simulink model "sampleModel291"  (R2021b)
settings: Solver=VariableStepAuto  StartTime=0.0  StopTime=10.0  RelTol=1e-3
undefined symbols (not defined in the file or in its folder): DiscIntNeverNeededParam
libraries: simulink x16, slpidlib x3
settings Model: Creator=user  LastModifiedBy=user

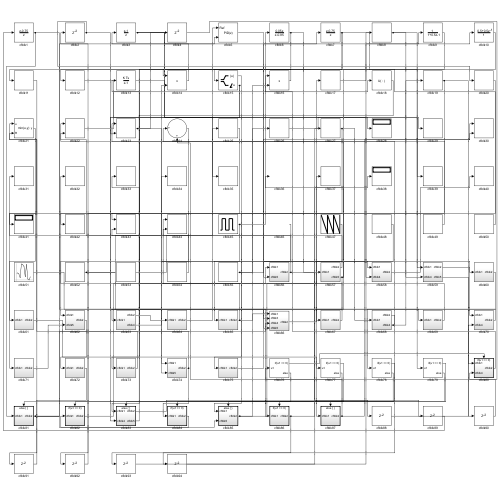
[thumbnail: Simulink's stored preview of the top-level diagram]
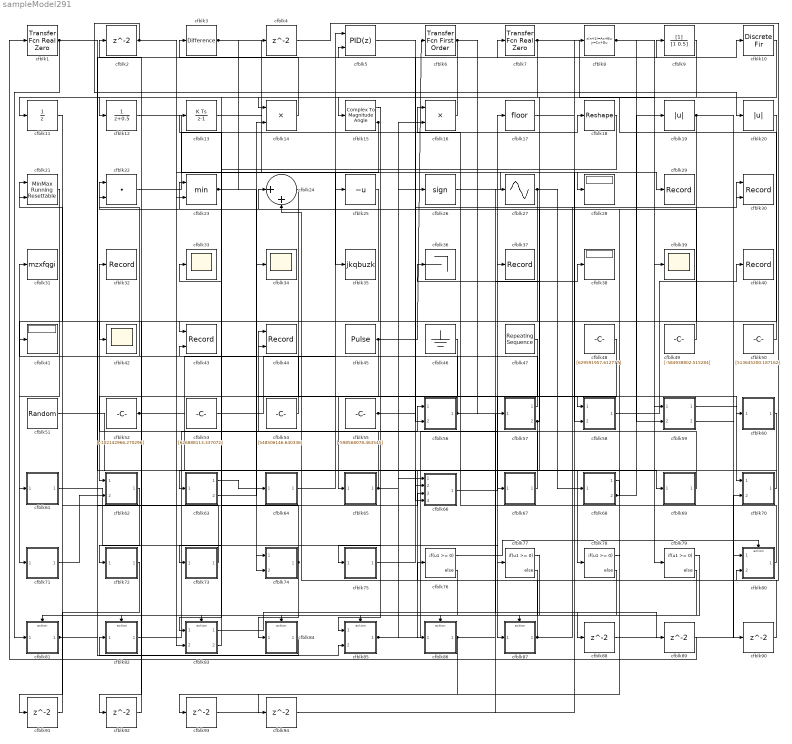
== system sampleModel291 ==
  cfblk1 : simulink/Discrete/Transfer Fcn Real Zero  ZeroZ=0.75  ICPrevInput=0.0  DoSatur=off
      settings: SourceProductBaseCode=SL
  cfblk10 : DiscreteFir  SampleTime=1
  cfblk11 : UnitDelay  HasFrameUpgradeWarning=on
  cfblk12 : DiscreteTransferFcn  SampleTime=1
  cfblk13 : DiscreteIntegrator  ICPrevOutput=DiscIntNeverNeededParam  ICPrevScaledInput=DiscIntNeverNeededParam
  cfblk14 : Product  Inputs=**
  cfblk15 : ComplexToMagnitudeAngle
  cfblk16 : Product
  cfblk17 : Rounding
  cfblk18 : Reshape
  cfblk19 : Abs
  cfblk{2,4,88..94} (9 alike) : Delay  SampleTime=1
  cfblk20 : Abs
  cfblk21 : simulink/Math Operations/MinMax Running Resettable  Function=min  vinit=0.0
  cfblk22 : DotProduct  InputSameDT=on  OutDataTypeStr=Inherit: Inherit via internal rule
  cfblk23 : MinMax  Inputs=2
  cfblk24 : Sum  Inputs=|++
  cfblk25 : UnaryMinus
  cfblk26 : Signum
  cfblk27 : Sin  TimeSource=Use external signal  SampleTime=0
  cfblk28 : Display
  cfblk29 : Record  FileSettingsInternal="{\"entries\":[{\"content\":{\"excelSettings\":{\"content\":{},\"type\":\"Streamout.ExcelSettings\"}},\"type\":\"Streamout.FileSettingStorage\",\"uuid\":\"2b0b6815-d365-4954-8dd6-cb2e8cf74314\"}],\"packageUris\":[\"http://schema.mathworks.com/mf0/streamout_blocks/R2020a\"],\"version\":\"1.0\"}"  SignalsInternal="{\"entries\":[{\"content\":{\"signals\":[{\"content\":{\"blockPath\":[\"sampleModel291/cfblk29\"],\"channel\":[],\"dimensions\":[1],\"domain\":\"sampleModel291/cfblk29\",\"lineColor\":\"#edb120\",\"plots\":[1],\"port\":1,\"sid\":[\"\"],\"signalID\":12456,\"signalName\":\"cfblk26\"},\"type\":\"RecordBlkView.Signal\",\"uuid\":\"788e08af-b9e6-414c-a560-80c9ba5d0819\"}]},\"type\":\"RecordBlkView.InputSignals\",\"uuid\":\"3e41c427-b0fd-42bd-a14a-d0577fb3f8b5\"}],\"packageUris\":[\"http://schema.mathworks.com/mf0/streamout_blocks/R2020a\"],\"version\":\"1.0\"}"  VisualizationBindings="{\"sparklinesplugin\":{\"info\":[{\"bindingParametersList\":[],\"subplotID\":1}]}}"
  cfblk3 : simulink/Discrete/Difference  ICPrevInput=0.0  OutMin=[]  OutMax=[]  OutDataTypeStr=Inherit: Inherit via back propagation  OutDataType=fixdt(1, 16)  OutScaling=2^-10  DoSatur=off
  cfblk30 : Record  FileSettingsInternal="{\"entries\":[{\"content\":{\"excelSettings\":{\"content\":{},\"type\":\"Streamout.ExcelSettings\"}},\"type\":\"Streamout.FileSettingStorage\",\"uuid\":\"5635bea9-fca3-4bb6-9632-28c56633b247\"}],\"packageUris\":[\"http://schema.mathworks.com/mf0/streamout_blocks/R2020a\"],\"version\":\"1.0\"}"  Layout=[1 1]  SignalsInternal="{\"entries\":[{\"content\":{\"signals\":[{\"content\":{\"blockPath\":[\"sampleModel291/cfblk30\"],\"channel\":[],\"dimensions\":[1],\"domain\":\"sampleModel291/cfblk30\",\"lineColor\":\"#a2142f\",\"plots\":[1],\"port\":1,\"sid\":[\"\"],\"signalID\":12460,\"signalName\":\"cfblk87\"},\"type\":\"RecordBlkView.Signal\",\"uuid\":\"f6ba7891-6f58-490e-8c31-e94127d30383\"},{\"content\":{\"blockPath\":[\"sampleModel291/cfblk30\"],\"channel\":[],\"dimensions\":[1],\"domain\":\"sampleModel291/cfblk30\",\"lineColor\":\"#139fff\",\"plots\":[1],\"port\":2,\"sid\":[\"\"],\"signalID\":12464,\"signalName\":\"cfblk55\"},\"type\":\"RecordBlkView.Signal\",\"uuid\":\"f8dfc05c-fd6f-41d1-b156-836e96f304bb\"}]},\"type\":\"RecordBlkView.InputSignals\",\"uuid\":\"be853f81-9516-4f72-8c0c-f98c43faa0f0\"}],\"packageUris\":[\"http://schema.mathworks.com/mf0/streamout_blocks/R2020a\"],\"version\":\"1.0\"}"  VisualizationBindings="{\"xyplotplugin\":{\"info\":[{\"series\":[{\"bindingParametersList\":[{\"parameter\":\"X-Axis\",\"signalID\":12460,\"signalName\":\"cfblk87\"},{\"parameter\":\"Y-Axis\",\"signalID\":12464,\"signalName\":\"cfblk55\"}],\"seriesID\":59280}],\"subplotID\":1}]}}"  CompatibilityTag=XY
  cfblk31 : ToWorkspace  VariableName=mzxfqgi  SaveFormat=Timeseries  SampleTime=-1
  cfblk32 : Record  FileSettingsInternal="{\"entries\":[{\"content\":{\"excelSettings\":{\"content\":{},\"type\":\"Streamout.ExcelSettings\"}},\"type\":\"Streamout.FileSettingStorage\",\"uuid\":\"60596596-cd23-4a4b-82c4-f6842354ffef\"}],\"packageUris\":[\"http://schema.mathworks.com/mf0/streamout_blocks/R2020a\"],\"version\":\"1.0\"}"  SignalsInternal="{\"entries\":[{\"content\":{\"signals\":[{\"content\":{\"blockPath\":[\"sampleModel291/cfblk32\"],\"channel\":[],\"dimensions\":[1],\"domain\":\"sampleModel291/cfblk32\",\"lineColor\":\"#4dbeee\",\"plots\":[1],\"port\":1,\"sid\":[\"\"],\"signalID\":12468,\"signalName\":\"cfblk69\"},\"type\":\"RecordBlkView.Signal\",\"uuid\":\"650ce02e-d49f-4bcf-a60e-c9fb45e201ce\"}]},\"type\":\"RecordBlkView.InputSignals\",\"uuid\":\"14e7f9b7-81f6-4e45-abef-a96e68b35e17\"}],\"packageUris\":[\"http://schema.mathworks.com/mf0/streamout_blocks/R2020a\"],\"version\":\"1.0\"}"  VisualizationBindings="{\"sparklinesplugin\":{\"info\":[{\"bindingParametersList\":[],\"subplotID\":1}]}}"
  cfblk{33..34,39,42} (4 alike) : Scope
  cfblk35 : ToWorkspace  VariableName=jkqbuzk  SaveFormat=Timeseries  SampleTime=-1
  cfblk36 : Terminator
  cfblk37 : Record  FileSettingsInternal="{\"entries\":[{\"content\":{\"excelSettings\":{\"content\":{},\"type\":\"Streamout.ExcelSettings\"}},\"type\":\"Streamout.FileSettingStorage\",\"uuid\":\"270472a9-c15e-4337-86cb-d1870147eddd\"}],\"packageUris\":[\"http://schema.mathworks.com/mf0/streamout_blocks/R2020a\"],\"version\":\"1.0\"}"  SignalsInternal="{\"entries\":[{\"content\":{\"signals\":[{\"content\":{\"blockPath\":[\"sampleModel291/cfblk37\"],\"channel\":[],\"dimensions\":[1],\"domain\":\"sampleModel291/cfblk37\",\"lineColor\":\"#a2142f\",\"plots\":[1],\"port\":1,\"sid\":[\"\"],\"signalID\":12472,\"signalName\":\"cfblk66\"},\"type\":\"RecordBlkView.Signal\",\"uuid\":\"8edad1df-9d97-4163-a96f-1843b3050bc3\"}]},\"type\":\"RecordBlkView.InputSignals\",\"uuid\":\"f9057b6f-5984-4fda-84d3-36f6257ae627\"}],\"packageUris\":[\"http://schema.mathworks.com/mf0/streamout_blocks/R2020a\"],\"version\":\"1.0\"}"  VisualizationBindings="{\"sparklinesplugin\":{\"info\":[{\"bindingParametersList\":[],\"subplotID\":1}]}}"
  cfblk38 : Display
  cfblk40 : Record  FileSettingsInternal="{\"entries\":[{\"content\":{\"excelSettings\":{\"content\":{},\"type\":\"Streamout.ExcelSettings\"}},\"type\":\"Streamout.FileSettingStorage\",\"uuid\":\"e3efeabe-4dc1-445f-9362-73d41ad3b046\"}],\"packageUris\":[\"http://schema.mathworks.com/mf0/streamout_blocks/R2020a\"],\"version\":\"1.0\"}"  SignalsInternal="{\"entries\":[{\"content\":{\"signals\":[{\"content\":{\"blockPath\":[\"sampleModel291/cfblk40\"],\"channel\":[],\"dimensions\":[1],\"domain\":\"sampleModel291/cfblk40\",\"lineColor\":\"#139fff\",\"plots\":[1],\"port\":1,\"sid\":[\"\"],\"signalID\":12476,\"signalName\":\"cfblk58\"},\"type\":\"RecordBlkView.Signal\",\"uuid\":\"9cd40f56-8516-48ae-bdeb-aa173b96d6b5\"}]},\"type\":\"RecordBlkView.InputSignals\",\"uuid\":\"edb59d7e-1718-46a5-85a3-ead406b706be\"}],\"packageUris\":[\"http://schema.mathworks.com/mf0/streamout_blocks/R2020a\"],\"version\":\"1.0\"}"  VisualizationBindings="{\"sparklinesplugin\":{\"info\":[{\"bindingParametersList\":[],\"subplotID\":1}]}}"
  cfblk41 : Display
  cfblk43 : Record  FileSettingsInternal="{\"entries\":[{\"content\":{\"excelSettings\":{\"content\":{},\"type\":\"Streamout.ExcelSettings\"}},\"type\":\"Streamout.FileSettingStorage\",\"uuid\":\"b99e1a35-57bf-4256-9eb8-cedfd4ac4627\"}],\"packageUris\":[\"http://schema.mathworks.com/mf0/streamout_blocks/R2020a\"],\"version\":\"1.0\"}"  Layout=[1 1]  SignalsInternal="{\"entries\":[{\"content\":{\"signals\":[{\"content\":{\"blockPath\":[\"sampleModel291/cfblk43\"],\"channel\":[],\"dimensions\":[1],\"domain\":\"sampleModel291/cfblk43\",\"lineColor\":\"#a2142f\",\"plots\":[1],\"port\":1,\"sid\":[\"\"],\"signalID\":12480,\"signalName\":\"cfblk18\"},\"type\":\"RecordBlkView.Signal\",\"uuid\":\"0c827c99-4b19-44af-998e-2d70f7f43936\"},{\"content\":{\"blockPath\":[\"sampleModel291/cfblk43\"],\"channel\":[],\"dimensions\":[1],\"domain\":\"sampleModel291/cfblk43\",\"lineColor\":\"#139fff\",\"plots\":[1],\"port\":2,\"sid\":[\"\"],\"signalID\":12484,\"signalName\":\"cfblk74\"},\"type\":\"RecordBlkView.Signal\",\"uuid\":\"e2180e44-affb-4eca-9fa8-177fe43e3fdb\"}]},\"type\":\"RecordBlkView.InputSignals\",\"uuid\":\"4fbe75a2-a5ef-434c-95ec-d27dfedd3f1a\"}],\"packageUris\":[\"http://schema.mathworks.com/mf0/streamout_blocks/R2020a\"],\"version\":\"1.0\"}"  VisualizationBindings="{\"xyplotplugin\":{\"info\":[{\"series\":[{\"bindingParametersList\":[{\"parameter\":\"X-Axis\",\"signalID\":12480,\"signalName\":\"cfblk18\"},{\"parameter\":\"Y-Axis\",\"signalID\":12484,\"signalName\":\"cfblk74\"}],\"seriesID\":65002}],\"subplotID\":1}]}}"  CompatibilityTag=XY
  cfblk44 : Record  FileSettingsInternal="{\"entries\":[{\"content\":{\"excelSettings\":{\"content\":{},\"type\":\"Streamout.ExcelSettings\"}},\"type\":\"Streamout.FileSettingStorage\",\"uuid\":\"dd3e8336-4d39-4557-9814-8ffac90a22b5\"}],\"packageUris\":[\"http://schema.mathworks.com/mf0/streamout_blocks/R2020a\"],\"version\":\"1.0\"}"  Layout=[1 1]  SignalsInternal="{\"entries\":[{\"content\":{\"signals\":[{\"content\":{\"blockPath\":[\"sampleModel291/cfblk44\"],\"channel\":[],\"dimensions\":[1],\"domain\":\"sampleModel291/cfblk44\",\"lineColor\":\"#a2142f\",\"plots\":[1],\"port\":1,\"sid\":[\"\"],\"signalID\":12488,\"signalName\":\"cfblk54\"},\"type\":\"RecordBlkView.Signal\",\"uuid\":\"f76f9e45-b488-469e-872e-e77342bc62c3\"},{\"content\":{\"blockPath\":[\"sampleModel291/cfblk44\"],\"channel\":[],\"dimensions\":[1],\"domain\":\"sampleModel291/cfblk44\",\"lineColor\":\"#139fff\",\"plots\":[1],\"port\":2,\"sid\":[\"\"],\"signalID\":12492,\"signalName\":\"cfblk67\"},\"type\":\"RecordBlkView.Signal\",\"uuid\":\"5a00877b-0bba-45c6-97db-c17559165956\"}]},\"type\":\"RecordBlkView.InputSignals\",\"uuid\":\"02471b0b-4fe3-4949-b75a-dd1ba1dc8109\"}],\"packageUris\":[\"http://schema.mathworks.com/mf0/streamout_blocks/R2020a\"],\"version\":\"1.0\"}"  VisualizationBindings="{\"xyplotplugin\":{\"info\":[{\"series\":[{\"bindingParametersList\":[{\"parameter\":\"X-Axis\",\"signalID\":12488,\"signalName\":\"cfblk54\"},{\"parameter\":\"Y-Axis\",\"signalID\":12492,\"signalName\":\"cfblk67\"}],\"seriesID\":5305}],\"subplotID\":1}]}}"  CompatibilityTag=XY
  cfblk45 : DiscretePulseGenerator  PulseType=Time based  Amplitude=[-963080004.086267]  Period=[93072844.377323]  PulseWidth=5  PhaseDelay=[6.000000]
  cfblk46 : Ground
  cfblk47 : simulink/Sources/Repeating Sequence  rep_seq_t=[0 2]  rep_seq_y=[783761546.915751, 763505204.571826]
  cfblk48 : Constant  Value=[629591957.612777]  SampleTime=1
  cfblk49 : Constant  Value=[-584938802.515284]  SampleTime=1
  cfblk5 : slpidlib/PID Controller (2DOF)  Controller=PID  Form=Parallel  TimeDomain=Discrete-time  UseExternalTs=off  SampleTime=1  IntegratorMethod=Forward Euler  FilterMethod=Forward Euler  ControllerParametersSource=internal  P=1  I=1  D=0  UseFilter=on  N=100  b=1  c=1  TunerSelectOption=Transfer Function Based (PID Tuner App)  InitialConditionSource=internal  InitialConditionForIntegrator=0  InitialConditionForFilter=0  DifferentiatorICPrevScaledInput=0  ExternalReset=none  TrackingMode=off  Kt=1  LimitOutput=off  SatLimitsSource=internal  UpperSaturationLimit=inf  LowerSaturationLimit=-inf  LinearizeAsGain=off  AntiWindupMode=none  Kb=1  POutMin=[]  POutMax=[]  IOutMin=[]  IOutMax=[]  DOutMin=[]  DOutMax=[]  NOutMin=[]  NOutMax=[]  bOutMin=[]  bOutMax=[]  cOutMin=[]  cOutMax=[]  SumOutMin=[]  SumOutMax=[]  SaturationOutMin=[]  SaturationOutMax=[]  PParamMin=[]  PParamMax=[]  IParamMin=[]  IParamMax=[]  DParamMin=[]  DParamMax=[]  NParamMin=[]  NParamMax=[]  bParamMin=[]  bParamMax=[]  cParamMin=[]  cParamMax=[]  KbParamMin=[]  KbParamMax=[]  KtParamMin=[]  KtParamMax=[]  KbOutMin=[]  KbOutMax=[]  KtOutMin=[]  KtOutMax=[]  IntegratorOutMin=[]  IntegratorOutMax=[]  FilterOutMin=[]  FilterOutMax=[]  SumI1OutMin=[]  SumI1OutMax=[]  SumI2OutMin=[]  SumI2OutMax=[]  SumI3OutMin=[]  SumI3OutMax=[]  SumI4OutMin=[]  SumI4OutMax=[]  SumDOutMin=[]  SumDOutMax=[]  Sum1OutMin=[]  Sum1OutMax=[]  Sum2OutMin=[]  Sum2OutMax=[]  Sum3OutMin=[]  Sum3OutMax=[]  DifferentiatorOutMin=[]  DifferentiatorOutMax=[]  FilterDiffOutCoefMin=[]  FilterDiffOutCoefMax=[]  ReciprocalOutMin=[]  ReciprocalOutMax=[]  SumDenOutMin=[]  SumDenOutMax=[]  SumNumOutMin=[]  SumNumOutMax=[]  DivideOutMin=[]  DivideOutMax=[]  UdiffTsProdOutMin=[]  UdiffTsProdOutMax=[]  NTsProdOutMin=[]  NTsProdOutMax=[]  UintegralTsProdOutMin=[]  UintegralTsProdOutMax=[]  UngainTsProdOutMin=[]  UngainTsProdOutMax=[]  IntegratorContinuousStateAttributes=''  IntegratorStateMustResolveToSignalObject=off  IntegratorRTWStateStorageClass=Auto  FilterContinuousStateAttributes=''  FilterStateMustResolveToSignalObject=off  FilterRTWStateStorageClass=Auto  ParallelPVariant=InternalParameters  IdealPVariant=Disabled  IVariant=InternalParameters  DVariant=InternalParameters  bVariant=InternalParameters  cVariant=InternalParameters  IntegratorVariant=Discrete  SatVariant=Disabled  AWVariant=Passthrough  PCopyVariant=Disabled  TRVariant=Disabled  FdbkBlocksVariant=Forward  IdealPFdbkVariant=Disabled  SatFdbkVariant=Disabled  DerivativeFilterVariant=ForwardEulerFilter  NVariant=InternalParameters  NCopyVariant=Disabled  FilterICVariant=InternalICsFilter  IntegratorICVariant=InternalICs  ExternalResetVariant=Disabled  TRSumVariant=Passthrough  SumFdbkVariant=Disabled  SumVariant=Sum_PID  TsampFilterVariant=InternalTs  TsampNgainVariant=Passthrough  TsampIntegralVariant=Passthrough  ExternalSaturationOutDataTypeStr=Inherit: Same as second input
      settings: SourceProductBaseCode=SL
  cfblk50 : Constant  Value=[513645200.187162]  SampleTime=1
  cfblk51 : RandomNumber  Mean=[34863.969112]  Variance=[79855.509002]  Seed=[176318592.000000]  SampleTime=0.1
  cfblk52 : Constant  Value=[-102142966.270296]  SampleTime=1
  cfblk53 : Constant  Value=[626888113.337072]  SampleTime=1
  cfblk54 : Constant  Value=[548506146.640336]  SampleTime=1
  cfblk55 : Constant  Value=[-598568078.463545]  SampleTime=1
  cfblk56 : Subsystem
  cfblk57 : Subsystem
  cfblk58 : Subsystem
  cfblk59 : Subsystem
  cfblk6 : simulink/Discrete/Transfer Fcn First Order  PoleZ=0.95  ICPrevOutput=0.0  DoSatur=off
  cfblk60 : Subsystem
  cfblk61 : Subsystem
  cfblk62 : Subsystem
  cfblk63 : Subsystem
  cfblk64 : Subsystem
  cfblk65 : Subsystem
  cfblk66 : Subsystem
  cfblk67 : Subsystem
  cfblk68 : Subsystem
  cfblk69 : Subsystem
  cfblk7 : simulink/Discrete/Transfer Fcn Real Zero  ZeroZ=0.75  ICPrevInput=0.0  DoSatur=off
      settings: SourceProductBaseCode=SL
  cfblk70 : Subsystem
  cfblk71 : Subsystem
  cfblk72 : Subsystem
  cfblk73 : Subsystem
  cfblk74 : Subsystem
  cfblk75 : Subsystem
  cfblk{76..79} (4 alike) : If  IfExpression=u1 >= 0  SampleTime=1
  cfblk8 : DiscreteStateSpace
  cfblk80 : Subsystem  TreatAsAtomicUnit=on
  cfblk81 : Subsystem  TreatAsAtomicUnit=on
  cfblk82 : Subsystem  TreatAsAtomicUnit=on
  cfblk83 : Subsystem  TreatAsAtomicUnit=on
  cfblk84 : Subsystem  TreatAsAtomicUnit=on
  cfblk85 : Subsystem  TreatAsAtomicUnit=on
  cfblk86 : Subsystem  TreatAsAtomicUnit=on
  cfblk87 : Subsystem  TreatAsAtomicUnit=on
  cfblk9 : DiscreteFilter  SampleTime=1
  wires:
  cfblk60/1(cfblk2) -> cfblk78/1
  cfblk22/1 -> cfblk18/1
  cfblk87/1(cfblk2) -> cfblk30/1, cfblk24/2
  cfblk63/1(cfblk2) -> cfblk64/1(cfblk1)
  cfblk24/1 -> cfblk62/1(cfblk1)
  cfblk84/1(cfblk2) -> cfblk82/1(cfblk1)
  cfblk82/1(cfblk2) -> cfblk56/1(cfblk1)
  cfblk50/1 -> cfblk11/1
  cfblk26/1 -> cfblk29/1
  cfblk16/1 -> cfblk12/1
  cfblk2/1 -> cfblk20/1, cfblk66/4(cfblk5)
  cfblk74/1(cfblk2) -> cfblk84/1(cfblk1), cfblk43/2
  cfblk18/1 -> cfblk43/1
  cfblk47/1 -> cfblk87/1(cfblk1)
  cfblk61/1(cfblk2) -> cfblk77/1
  cfblk12/1 -> cfblk28/1
  cfblk8/1 -> cfblk79/1, cfblk59/2(cfblk4)
  cfblk62/1(cfblk2) -> cfblk72/1(cfblk1)
  cfblk14/1 -> cfblk3/1
  cfblk85/1(cfblk2) -> cfblk17/1, cfblk16/2
  cfblk21/1 -> cfblk71/1(cfblk1)
  cfblk17/1 -> cfblk9/1
  cfblk57/1(cfblk2) -> cfblk31/1
  cfblk6/1 -> cfblk15/1, cfblk57/1(cfblk1)
  cfblk86/1(cfblk2) -> cfblk38/1, cfblk93/1
  cfblk19/1 -> cfblk80/1(cfblk1), cfblk42/1
  cfblk7/1 -> cfblk39/1, cfblk14/1, cfblk73/1(cfblk1)
  cfblk57/2(cfblk5) -> cfblk22/1, cfblk36/1, cfblk66/2(cfblk3)
  cfblk54/1 -> cfblk44/1
  cfblk65/1(cfblk2) -> cfblk33/1, cfblk66/1(cfblk1)
  cfblk66/1(cfblk2) -> cfblk37/1
  cfblk67/1(cfblk2) -> cfblk44/2
  cfblk53/1 -> cfblk5/1
  cfblk52/1 -> cfblk74/1(cfblk1), cfblk14/2
  cfblk49/1 -> cfblk23/1
  cfblk59/1(cfblk2) -> cfblk70/1(cfblk1)
  cfblk4/1 -> cfblk80/2(cfblk4)
  cfblk71/1(cfblk2) -> cfblk62/2(cfblk5)
  cfblk69/1(cfblk2) -> cfblk32/1
  cfblk46/1 -> cfblk65/1(cfblk1)
  cfblk1/1 -> cfblk81/1(cfblk1), cfblk69/1(cfblk1)
  cfblk56/1(cfblk2) -> cfblk22/2, cfblk88/1
  cfblk27/1 -> cfblk75/1(cfblk1), cfblk68/1(cfblk1)
  cfblk51/1 -> cfblk86/1(cfblk1)
  cfblk45/1 -> cfblk6/1, cfblk74/2(cfblk5)
  cfblk58/1(cfblk2) -> cfblk40/1
  cfblk15/1 -> cfblk85/1(cfblk1)
  cfblk70/1(cfblk2) -> cfblk63/1(cfblk1)
  cfblk5/1 -> cfblk60/1(cfblk1)
  cfblk64/1(cfblk2) -> cfblk25/1
  cfblk63/2(cfblk4) -> cfblk34/1
  cfblk80/1(cfblk2) -> cfblk16/1
  cfblk68/2(cfblk4) -> cfblk24/1, cfblk19/1
  cfblk73/1(cfblk2) -> cfblk21/1
  cfblk3/1 -> cfblk59/1(cfblk1), cfblk35/1, cfblk5/2
  cfblk48/1 -> cfblk56/2(cfblk5)
  cfblk25/1 -> cfblk61/1(cfblk1)
  cfblk23/1 -> cfblk58/1(cfblk1), cfblk4/1
  cfblk13/1 -> cfblk58/2(cfblk4)
  cfblk81/1(cfblk2) -> cfblk7/1, cfblk85/2(cfblk5), cfblk66/3(cfblk4)
  cfblk9/1 -> cfblk83/1(cfblk1)
  cfblk55/1 -> cfblk30/2, cfblk26/1
  cfblk75/1(cfblk2) -> cfblk10/1
  cfblk11/1 -> cfblk41/1
  cfblk83/2(cfblk5) -> cfblk13/1
  cfblk15/2 -> cfblk23/2, cfblk83/2(cfblk4)
  cfblk10/1 -> cfblk67/1(cfblk1)
  cfblk76/1 -> cfblk80/Action
  cfblk76/2 -> cfblk81/Action
  cfblk77/1 -> cfblk82/Action
  cfblk77/2 -> cfblk83/Action
  cfblk78/1 -> cfblk84/Action
  cfblk78/2 -> cfblk85/Action
  cfblk79/1 -> cfblk86/Action
  cfblk79/2 -> cfblk87/Action
  cfblk88/1 -> cfblk70/2(cfblk4)
  cfblk83/1(cfblk2) -> cfblk89/1
  cfblk89/1 -> cfblk1/1
  cfblk59/2(cfblk5) -> cfblk90/1
  cfblk90/1 -> cfblk76/1
  cfblk72/1(cfblk2) -> cfblk91/1
  cfblk91/1 -> cfblk21/2
  cfblk20/1 -> cfblk92/1
  cfblk92/1 -> cfblk2/1
  cfblk93/1 -> cfblk8/1
  cfblk68/1(cfblk2) -> cfblk94/1
  cfblk94/1 -> cfblk27/1

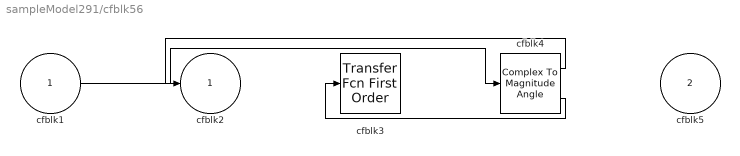
== system sampleModel291/cfblk56 ==
  cfblk1 : Inport
  cfblk5 : Inport  Port=2
  cfblk3 : simulink/Discrete/Transfer Fcn First Order  PoleZ=0.95  ICPrevOutput=0.0  DoSatur=off
  cfblk4 : ComplexToMagnitudeAngle
  cfblk2 : Outport
  wires:
  cfblk1/1 -> cfblk4/1
  cfblk4/1 -> cfblk2/1
  cfblk4/2 -> cfblk3/1

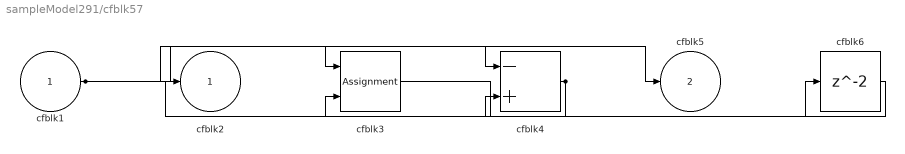
== system sampleModel291/cfblk57 ==
  cfblk1 : Inport
  cfblk3 : Assignment  DiagnosticForDimensions=Warning  IndexOptions=Index vector (dialog)  Indices=1  OutputSizes=1
  cfblk4 : Sum  Inputs=-+
  cfblk6 : Delay  SampleTime=1
  cfblk2 : Outport
  cfblk5 : Outport  Port=2
  wires:
  cfblk1/1 -> cfblk4/1, cfblk5/1, cfblk3/1
  cfblk4/1 -> cfblk2/1, cfblk3/2
  cfblk3/1 -> cfblk6/1
  cfblk6/1 -> cfblk4/2

== system sampleModel291/cfblk58 ==
  cfblk1 : Inport
  cfblk4 : Inport  Port=2
  cfblk3 : DiscreteFir  SampleTime=1
  cfblk2 : Outport
  wires:
  cfblk1/1 -> cfblk2/1
  cfblk4/1 -> cfblk3/1

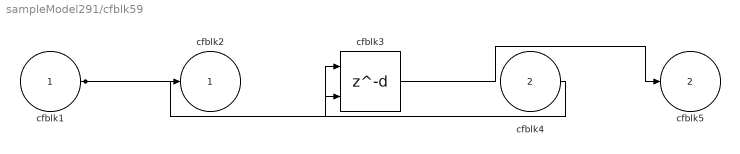
== system sampleModel291/cfblk59 ==
  cfblk1 : Inport
  cfblk4 : Inport  Port=2
  cfblk3 : Delay  DelayLengthSource=Input port  SampleTime=1
      settings: InputPortMap=u0,p1
  cfblk2 : Outport
  cfblk5 : Outport  Port=2
  wires:
  cfblk3/1 -> cfblk5/1
  cfblk4/1 -> cfblk3/1
  cfblk1/1 -> cfblk3/2, cfblk2/1

== system sampleModel291/cfblk60 ==
  cfblk1 : Inport
  cfblk3 : simulink/Discrete/Transfer Fcn First Order  PoleZ=0.95  ICPrevOutput=0.0  DoSatur=off
  cfblk4 : slpidlib/PID Controller  Controller=PID  Form=Parallel  TimeDomain=Discrete-time  UseExternalTs=off  SampleTime=1  IntegratorMethod=Forward Euler  FilterMethod=Forward Euler  ControllerParametersSource=internal  P=1  I=1  D=0  UseFilter=on  N=100  TunerSelectOption=Transfer Function Based (PID Tuner App)  InitialConditionSource=internal  InitialConditionForIntegrator=0  InitialConditionForFilter=0  DifferentiatorICPrevScaledInput=0  ExternalReset=none  TrackingMode=off  Kt=1  LimitOutput=off  SatLimitsSource=internal  UpperSaturationLimit=inf  LowerSaturationLimit=-inf  LinearizeAsGain=off  AntiWindupMode=none  Kb=1  POutMin=[]  POutMax=[]  IOutMin=[]  IOutMax=[]  DOutMin=[]  DOutMax=[]  NOutMin=[]  NOutMax=[]  SumOutMin=[]  SumOutMax=[]  SaturationOutMin=[]  SaturationOutMax=[]  PParamMin=[]  PParamMax=[]  IParamMin=[]  IParamMax=[]  DParamMin=[]  DParamMax=[]  NParamMin=[]  NParamMax=[]  KbParamMin=[]  KbParamMax=[]  KtParamMin=[]  KtParamMax=[]  KbOutMin=[]  KbOutMax=[]  KtOutMin=[]  KtOutMax=[]  IntegratorOutMin=[]  IntegratorOutMax=[]  FilterOutMin=[]  FilterOutMax=[]  SumI1OutMin=[]  SumI1OutMax=[]  SumI2OutMin=[]  SumI2OutMax=[]  SumI3OutMin=[]  SumI3OutMax=[]  SumI4OutMin=[]  SumI4OutMax=[]  SumDOutMin=[]  SumDOutMax=[]  DifferentiatorOutMin=[]  DifferentiatorOutMax=[]  FilterDiffOutCoefMin=[]  FilterDiffOutCoefMax=[]  ReciprocalOutMin=[]  ReciprocalOutMax=[]  SumDenOutMin=[]  SumDenOutMax=[]  SumNumOutMin=[]  SumNumOutMax=[]  DivideOutMin=[]  DivideOutMax=[]  UdiffTsProdOutMin=[]  UdiffTsProdOutMax=[]  NTsProdOutMin=[]  NTsProdOutMax=[]  UintegralTsProdOutMin=[]  UintegralTsProdOutMax=[]  UngainTsProdOutMin=[]  UngainTsProdOutMax=[]  IntegratorContinuousStateAttributes=''  IntegratorStateMustResolveToSignalObject=off  IntegratorRTWStateStorageClass=Auto  FilterContinuousStateAttributes=''  FilterStateMustResolveToSignalObject=off  FilterRTWStateStorageClass=Auto  ParallelPVariant=InternalParameters  IdealPVariant=Disabled  IVariant=InternalParameters  DVariant=InternalParameters  IntegratorVariant=Discrete  SatVariant=Disabled  AWVariant=Passthrough  PCopyVariant=Disabled  TRVariant=Disabled  FdbkBlocksVariant=Forward  IdealPFdbkVariant=Disabled  SatFdbkVariant=Disabled  DerivativeFilterVariant=ForwardEulerFilter  NVariant=InternalParameters  NCopyVariant=Disabled  FilterICVariant=InternalICsFilter  IntegratorICVariant=InternalICs  ExternalResetVariant=Disabled  TRSumVariant=Passthrough  SumFdbkVariant=Disabled  SumVariant=Sum_PID  TsampFilterVariant=InternalTs  TsampNgainVariant=Passthrough  TsampIntegralVariant=Passthrough  ExternalSaturationOutDataTypeStr=Inherit: Same as second input
  cfblk2 : Outport
  wires:
  cfblk1/1 -> cfblk3/1
  cfblk3/1 -> cfblk4/1
  cfblk4/1 -> cfblk2/1

== system sampleModel291/cfblk61 ==
  cfblk1 : Inport
  cfblk3 : Delay  SampleTime=1
  cfblk4 : simulink/Discrete/Transfer Fcn Real Zero  ZeroZ=0.75  ICPrevInput=0.0  DoSatur=off
      settings: SourceProductBaseCode=SL
  cfblk2 : Outport
  wires:
  cfblk1/1 -> cfblk4/1
  cfblk3/1 -> cfblk2/1
  cfblk4/1 -> cfblk3/1

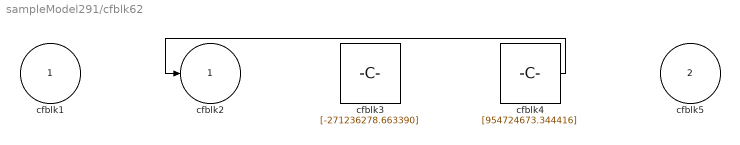
== system sampleModel291/cfblk62 ==
  cfblk1 : Inport
  cfblk5 : Inport  Port=2
  cfblk3 : Constant  Value=[-271236278.663390]  SampleTime=1
  cfblk4 : Constant  Value=[954724673.344416]  SampleTime=1
  cfblk2 : Outport
  wires:
  cfblk4/1 -> cfblk2/1

== system sampleModel291/cfblk63 ==
  cfblk1 : Inport
  cfblk3 : Constant  Value=[-201638452.809249]  SampleTime=1
  cfblk2 : Outport
  cfblk4 : Outport  Port=2
  wires:
  cfblk3/1 -> cfblk4/1
  cfblk1/1 -> cfblk2/1

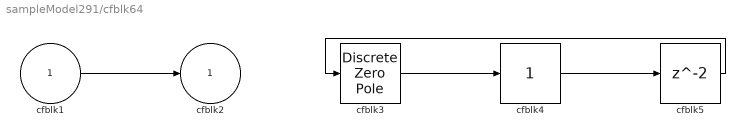
== system sampleModel291/cfblk64 ==
  cfblk1 : Inport
  cfblk3 : DiscreteZeroPole  Poles=[0 0.5]  Gain=1
  cfblk4 : simulink/Math Operations/Slider Gain  gain=1  low=0  high=2
  cfblk5 : Delay  SampleTime=1
  cfblk2 : Outport
  wires:
  cfblk3/1 -> cfblk4/1
  cfblk1/1 -> cfblk2/1
  cfblk4/1 -> cfblk5/1
  cfblk5/1 -> cfblk3/1

== system sampleModel291/cfblk65 ==
  cfblk1 : Inport
  cfblk3 : slpidlib/PID Controller (2DOF)  Controller=PID  Form=Parallel  TimeDomain=Discrete-time  UseExternalTs=off  SampleTime=1  IntegratorMethod=Forward Euler  FilterMethod=Forward Euler  ControllerParametersSource=internal  P=1  I=1  D=0  UseFilter=on  N=100  b=1  c=1  TunerSelectOption=Transfer Function Based (PID Tuner App)  InitialConditionSource=internal  InitialConditionForIntegrator=0  InitialConditionForFilter=0  DifferentiatorICPrevScaledInput=0  ExternalReset=none  TrackingMode=off  Kt=1  LimitOutput=off  SatLimitsSource=internal  UpperSaturationLimit=inf  LowerSaturationLimit=-inf  LinearizeAsGain=off  AntiWindupMode=none  Kb=1  POutMin=[]  POutMax=[]  IOutMin=[]  IOutMax=[]  DOutMin=[]  DOutMax=[]  NOutMin=[]  NOutMax=[]  bOutMin=[]  bOutMax=[]  cOutMin=[]  cOutMax=[]  SumOutMin=[]  SumOutMax=[]  SaturationOutMin=[]  SaturationOutMax=[]  PParamMin=[]  PParamMax=[]  IParamMin=[]  IParamMax=[]  DParamMin=[]  DParamMax=[]  NParamMin=[]  NParamMax=[]  bParamMin=[]  bParamMax=[]  cParamMin=[]  cParamMax=[]  KbParamMin=[]  KbParamMax=[]  KtParamMin=[]  KtParamMax=[]  KbOutMin=[]  KbOutMax=[]  KtOutMin=[]  KtOutMax=[]  IntegratorOutMin=[]  IntegratorOutMax=[]  FilterOutMin=[]  FilterOutMax=[]  SumI1OutMin=[]  SumI1OutMax=[]  SumI2OutMin=[]  SumI2OutMax=[]  SumI3OutMin=[]  SumI3OutMax=[]  SumI4OutMin=[]  SumI4OutMax=[]  SumDOutMin=[]  SumDOutMax=[]  Sum1OutMin=[]  Sum1OutMax=[]  Sum2OutMin=[]  Sum2OutMax=[]  Sum3OutMin=[]  Sum3OutMax=[]  DifferentiatorOutMin=[]  DifferentiatorOutMax=[]  FilterDiffOutCoefMin=[]  FilterDiffOutCoefMax=[]  ReciprocalOutMin=[]  ReciprocalOutMax=[]  SumDenOutMin=[]  SumDenOutMax=[]  SumNumOutMin=[]  SumNumOutMax=[]  DivideOutMin=[]  DivideOutMax=[]  UdiffTsProdOutMin=[]  UdiffTsProdOutMax=[]  NTsProdOutMin=[]  NTsProdOutMax=[]  UintegralTsProdOutMin=[]  UintegralTsProdOutMax=[]  UngainTsProdOutMin=[]  UngainTsProdOutMax=[]  IntegratorContinuousStateAttributes=''  IntegratorStateMustResolveToSignalObject=off  IntegratorRTWStateStorageClass=Auto  FilterContinuousStateAttributes=''  FilterStateMustResolveToSignalObject=off  FilterRTWStateStorageClass=Auto  ParallelPVariant=InternalParameters  IdealPVariant=Disabled  IVariant=InternalParameters  DVariant=InternalParameters  bVariant=InternalParameters  cVariant=InternalParameters  IntegratorVariant=Discrete  SatVariant=Disabled  AWVariant=Passthrough  PCopyVariant=Disabled  TRVariant=Disabled  FdbkBlocksVariant=Forward  IdealPFdbkVariant=Disabled  SatFdbkVariant=Disabled  DerivativeFilterVariant=ForwardEulerFilter  NVariant=InternalParameters  NCopyVariant=Disabled  FilterICVariant=InternalICsFilter  IntegratorICVariant=InternalICs  ExternalResetVariant=Disabled  TRSumVariant=Passthrough  SumFdbkVariant=Disabled  SumVariant=Sum_PID  TsampFilterVariant=InternalTs  TsampNgainVariant=Passthrough  TsampIntegralVariant=Passthrough  ExternalSaturationOutDataTypeStr=Inherit: Same as second input
      settings: SourceProductBaseCode=SL
  cfblk4 : simulink/Math Operations/MinMax Running Resettable  Function=min  vinit=0.0
  cfblk2 : Outport
  wires:
  cfblk4/1 -> cfblk3/1
  cfblk1/1 -> cfblk3/2, cfblk4/1, cfblk4/2
  cfblk3/1 -> cfblk2/1

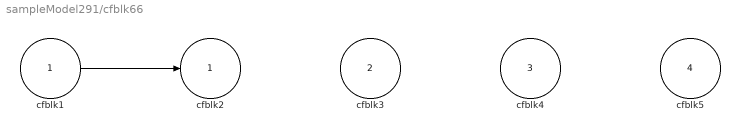
== system sampleModel291/cfblk66 ==
  cfblk1 : Inport
  cfblk3 : Inport  Port=2
  cfblk4 : Inport  Port=3
  cfblk5 : Inport  Port=4
  cfblk2 : Outport
  wires:
  cfblk1/1 -> cfblk2/1

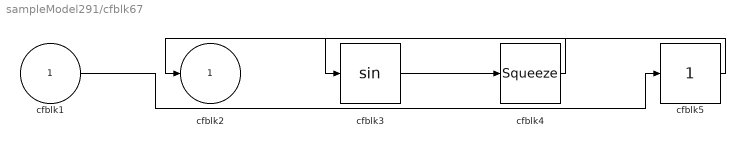
== system sampleModel291/cfblk67 ==
  cfblk1 : Inport
  cfblk3 : Trigonometry
  cfblk4 : Squeeze
  cfblk5 : simulink/Math Operations/Slider Gain  gain=1  low=0  high=2
  cfblk2 : Outport
  wires:
  cfblk4/1 -> cfblk2/1
  cfblk1/1 -> cfblk5/1
  cfblk3/1 -> cfblk4/1
  cfblk5/1 -> cfblk3/1

== system sampleModel291/cfblk68 ==
  cfblk1 : Inport
  cfblk3 : Math  Operator=pow  SaturateOnIntegerOverflow=on
  cfblk2 : Outport
  cfblk4 : Outport  Port=2
  wires:
  cfblk1/1 -> cfblk4/1, cfblk3/1, cfblk3/2
  cfblk3/1 -> cfblk2/1

== system sampleModel291/cfblk69 ==
  cfblk1 : Inport
  cfblk3 : simulink/Discrete/Transfer Fcn First Order  PoleZ=0.95  ICPrevOutput=0.0  DoSatur=off
  cfblk4 : PermuteDimensions
  cfblk5 : ComplexToMagnitudeAngle
  cfblk2 : Outport
  wires:
  cfblk5/1 -> cfblk2/1
  cfblk3/1 -> cfblk5/1
  cfblk5/2 -> cfblk4/1
  cfblk1/1 -> cfblk3/1

== system sampleModel291/cfblk70 ==
  cfblk1 : Inport
  cfblk4 : Inport  Port=2
  cfblk3 : Math  Operator=rem  SaturateOnIntegerOverflow=on
  cfblk2 : Outport
  wires:
  cfblk1/1 -> cfblk3/1
  cfblk4/1 -> cfblk3/2
  cfblk3/1 -> cfblk2/1

== system sampleModel291/cfblk71 ==
  cfblk1 : Inport
  cfblk3 : simulink/Discrete/Transfer Fcn First Order  PoleZ=0.95  ICPrevOutput=0.0  DoSatur=off
  cfblk2 : Outport
  wires:
  cfblk3/1 -> cfblk2/1
  cfblk1/1 -> cfblk3/1

== system sampleModel291/cfblk72 ==
  cfblk1 : Inport
  cfblk3 : Delay  DelayLengthSource=Input port  SampleTime=1
      settings: InputPortMap=u0,p1
  cfblk2 : Outport
  wires:
  cfblk1/1 -> cfblk3/1, cfblk3/2
  cfblk3/1 -> cfblk2/1

== system sampleModel291/cfblk73 ==
  cfblk1 : Inport
  cfblk3 : Trigonometry
  cfblk2 : Outport
  wires:
  cfblk1/1 -> cfblk2/1, cfblk3/1

== system sampleModel291/cfblk74 ==
  cfblk1 : Inport
  cfblk5 : Inport  Port=2
  cfblk3 : Sqrt  SaturateOnIntegerOverflow=on
  cfblk4 : Gain  Gain=[-474978337.652932]
  cfblk2 : Outport
  wires:
  cfblk1/1 -> cfblk4/1
  cfblk5/1 -> cfblk2/1
  cfblk4/1 -> cfblk3/1

== system sampleModel291/cfblk75 ==
  cfblk1 : Inport
  cfblk3 : Assignment  DiagnosticForDimensions=Warning  IndexOptions=Index vector (dialog)  Indices=1  OutputSizes=1
  cfblk4 : Abs
  cfblk2 : Outport
  wires:
  cfblk1/1 -> cfblk4/1
  cfblk4/1 -> cfblk2/1, cfblk3/1, cfblk3/2

== system sampleModel291/cfblk80 ==
  cfblk1 : Inport
  cfblk4 : Inport  Port=2
  Action Port : ActionPort  ActionPortLabel=if(u1 >= 0)
  cfblk3 : MinMax  Function=max  Inputs=3
  cfblk2 : Outport
  wires:
  cfblk3/1 -> cfblk2/1
  cfblk4/1 -> cfblk3/1, cfblk3/3
  cfblk1/1 -> cfblk3/2

== system sampleModel291/cfblk81 ==
  cfblk1 : Inport
  Action Port : ActionPort  ActionPortLabel=else
  cfblk3 : Signum
  cfblk2 : Outport
  wires:
  cfblk3/1 -> cfblk2/1
  cfblk1/1 -> cfblk3/1

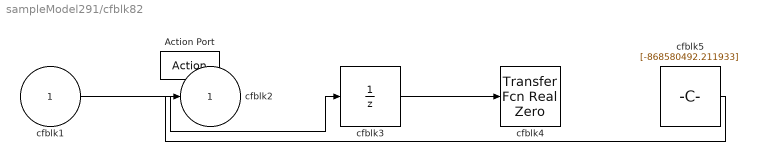
== system sampleModel291/cfblk82 ==
  cfblk1 : Inport
  Action Port : ActionPort  ActionPortLabel=if(u1 >= 0)
  cfblk3 : UnitDelay  SampleTime=-1  HasFrameUpgradeWarning=on
  cfblk4 : simulink/Discrete/Transfer Fcn Real Zero  ZeroZ=0.75  ICPrevInput=0.0  DoSatur=off
      settings: SourceProductBaseCode=SL
  cfblk5 : Constant  Value=[-868580492.211933]  SampleTime=1
  cfblk2 : Outport
  wires:
  cfblk1/1 -> cfblk3/1
  cfblk3/1 -> cfblk4/1
  cfblk5/1 -> cfblk2/1

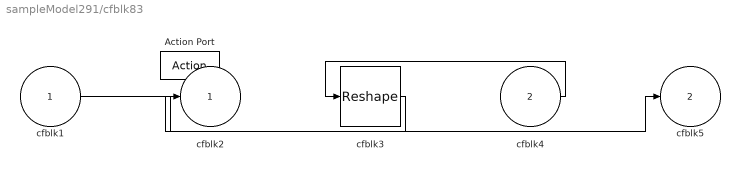
== system sampleModel291/cfblk83 ==
  cfblk1 : Inport
  cfblk4 : Inport  Port=2
  Action Port : ActionPort  ActionPortLabel=else
  cfblk3 : Reshape
  cfblk2 : Outport
  cfblk5 : Outport  Port=2
  wires:
  cfblk4/1 -> cfblk3/1
  cfblk1/1 -> cfblk5/1
  cfblk3/1 -> cfblk2/1

== system sampleModel291/cfblk84 ==
  cfblk1 : Inport
  Action Port : ActionPort  ActionPortLabel=if(u1 >= 0)
  cfblk3 : DotProduct  InputSameDT=on  OutDataTypeStr=Inherit: Inherit via internal rule
  cfblk2 : Outport
  wires:
  cfblk3/1 -> cfblk2/1
  cfblk1/1 -> cfblk3/1, cfblk3/2

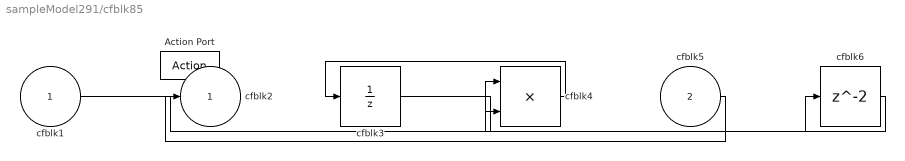
== system sampleModel291/cfblk85 ==
  cfblk1 : Inport
  cfblk5 : Inport  Port=2
  Action Port : ActionPort  ActionPortLabel=else
  cfblk3 : UnitDelay  SampleTime=-1  HasFrameUpgradeWarning=on
  cfblk4 : Product  Inputs=**
  cfblk6 : Delay
  cfblk2 : Outport
  wires:
  cfblk1/1 -> cfblk4/1
  cfblk5/1 -> cfblk2/1
  cfblk4/1 -> cfblk3/1
  cfblk3/1 -> cfblk6/1
  cfblk6/1 -> cfblk4/2

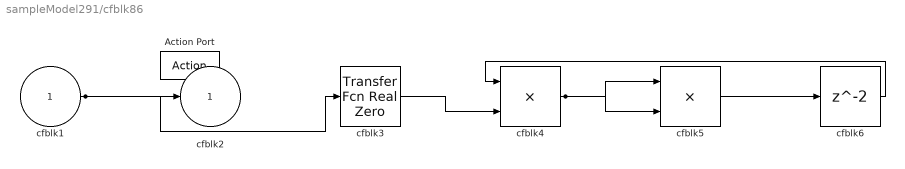
== system sampleModel291/cfblk86 ==
  cfblk1 : Inport
  Action Port : ActionPort  ActionPortLabel=if(u1 >= 0)
  cfblk3 : simulink/Discrete/Transfer Fcn Real Zero  ZeroZ=0.75  ICPrevInput=0.0  DoSatur=off
      settings: SourceProductBaseCode=SL
  cfblk4 : Product  Inputs=**
  cfblk5 : Product
  cfblk6 : Delay
  cfblk2 : Outport
  wires:
  cfblk1/1 -> cfblk2/1, cfblk3/1
  cfblk3/1 -> cfblk4/2
  cfblk4/1 -> cfblk5/1, cfblk5/2
  cfblk5/1 -> cfblk6/1
  cfblk6/1 -> cfblk4/1

== system sampleModel291/cfblk87 ==
  cfblk1 : Inport
  Action Port : ActionPort  ActionPortLabel=else
  cfblk3 : Assignment  DiagnosticForDimensions=Warning  IndexOptions=Index vector (dialog)  Indices=1  OutputSizes=1
  cfblk2 : Outport
  wires:
  cfblk1/1 -> cfblk3/1, cfblk3/2
  cfblk3/1 -> cfblk2/1
